simulink model "PurePuersuit"  (R2023a)
settings: Solver=VariableStepAuto  StartTime=0.0  StopTime=10.0  RelTol=1e-3
settings Model: Creator=余嘉乐  LastModifiedBy=余嘉乐

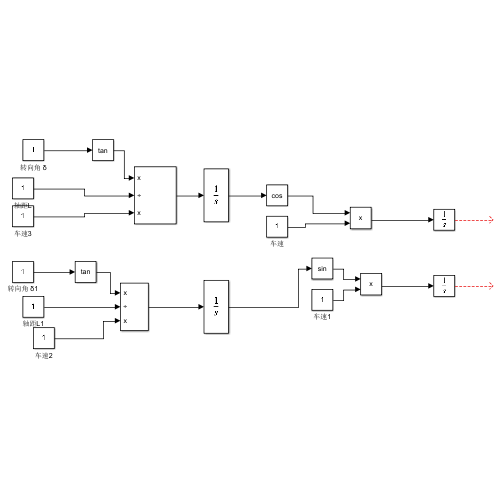
[thumbnail: Simulink's stored preview of the top-level diagram]
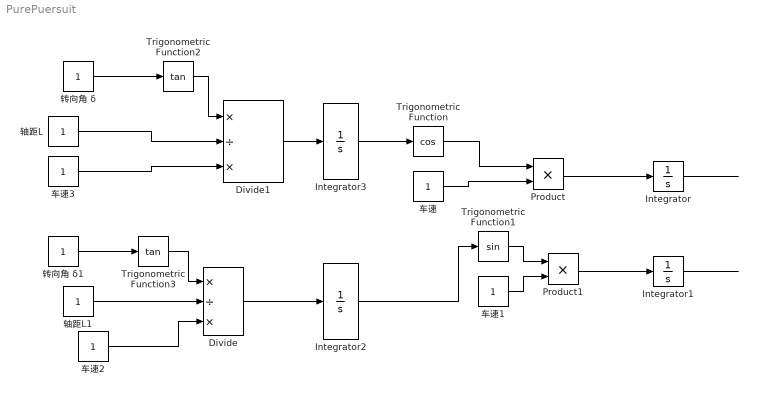
== system PurePuersuit ==
  Divide : Product  Inputs=*/*
  Divide1 : Product  Inputs=*/*
  Integrator{,1..3} (4 alike) : Integrator
  Product : Product
  Product1 : Product
  Trigonometric Function : Trigonometry  Operator=cos
  Trigonometric Function1 : Trigonometry
  Trigonometric Function2 : Trigonometry  Operator=tan
  Trigonometric Function3 : Trigonometry  Operator=tan
  车速{,1..3} (4 alike) : Constant
  转向角 δ : Constant
  转向角 δ1 : Constant
  轴距L : Constant
  轴距L1 : Constant
  wires:
  Trigonometric Function/1 -> Product/1
  车速/1 -> Product/2
  Product/1 -> Integrator/1
  Trigonometric Function1/1 -> Product1/1
  车速1/1 -> Product1/2
  Product1/1 -> Integrator1/1
  转向角 δ/1 -> Trigonometric Function2/1
  Trigonometric Function2/1 -> Divide1/1
  转向角 δ1/1 -> Trigonometric Function3/1
  Trigonometric Function3/1 -> Divide/1
  车速2/1 -> Divide/3
  Divide1/1 -> Integrator3/1
  车速3/1 -> Divide1/3
  轴距L/1 -> Divide1/2
  轴距L1/1 -> Divide/2
  Divide/1 -> Integrator2/1
  Integrator2/1 -> Trigonometric Function1/1
  Integrator3/1 -> Trigonometric Function/1
  Integrator/1 -> ?
  Integrator1/1 -> ?
